simulink model "s0311_Bayesopt_SimulatorParameters"  (R2019b)
settings: Solver=FixedStepAuto  StartTime=0.0  StopTime=T_sim  FixedStep=dt  RelTol=1e-3
settings Model: Creator=paolo  LastModifiedBy=giaco
settings DebuggingCC: SFMachineParentedDataDiag=error

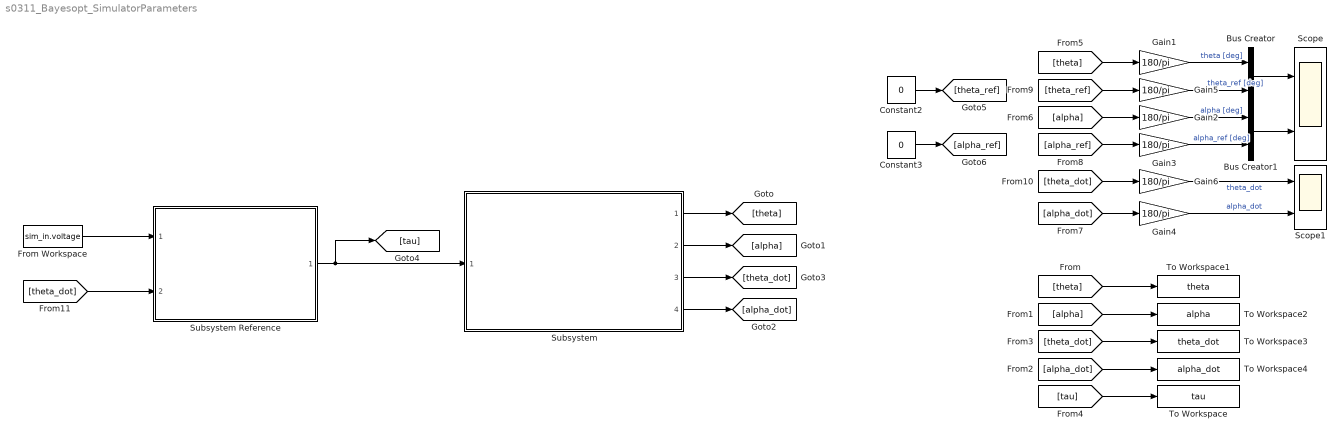
== system s0311_Bayesopt_SimulatorParameters ==
  Bus Creator : BusCreator  Inputs=2
  Bus Creator1 : BusCreator  Inputs=2
  Constant2 : Constant  Value=0
  Constant3 : Constant  Value=0
  From Workspace : FromWorkspace  VariableName=sim_in.voltage  SampleTime=0
  Gain{1..6} (6 alike) : Gain  Gain=180/pi
  Scope : Scope  NumInputPorts=2
  Scope1 : Scope  NumInputPorts=2
  Subsystem : Subsystem  ReferencedSubsystem=s0311_bayesopt_simulator  th_0=PARAMS.th_0  al_0=PARAMS.al_0  th_dot_0=PARAMS.th_dot_0  al_dot_0=PARAMS.al_dot_0
  Subsystem Reference : Subsystem  ReferencedSubsystem=s0303_motor_simulator  omega_0=PARAMS.th_dot_0  i_0=0
  To Workspace : ToWorkspace  VariableName=tau  SampleTime=-1
  To Workspace1 : ToWorkspace  VariableName=theta  SampleTime=-1
  To Workspace2 : ToWorkspace  VariableName=alpha  SampleTime=-1
  To Workspace3 : ToWorkspace  VariableName=theta_dot  SampleTime=-1
  To Workspace4 : ToWorkspace  VariableName=alpha_dot  SampleTime=-1
  wires:
  Subsystem/1 -> [theta]
  Subsystem/2 -> [alpha]
  Subsystem/4 -> [alpha_dot]
  Subsystem/3 -> [theta_dot]
  Subsystem Reference/1 -> Subsystem/1, [tau]
  From Workspace/1 -> Subsystem Reference/1
  [tau] -> To Workspace/1
  [theta] -> To Workspace1/1
  [alpha] -> To Workspace2/1
  [theta_dot] -> To Workspace3/1
  [alpha_dot] -> To Workspace4/1
  [theta] -> Gain1/1
  [alpha] -> Gain2/1
  [alpha_ref] -> Gain3/1
  [alpha_dot] -> Gain4/1
  Gain1/1 -> Bus Creator/1  "theta [deg]"
  [theta_ref] -> Gain5/1
  Gain5/1 -> Bus Creator/2  "theta_ref [deg]"
  Gain2/1 -> Bus Creator1/1  "alpha [deg]"
  Gain3/1 -> Bus Creator1/2  "alpha_ref [deg]"
  Constant2/1 -> [theta_ref]
  Constant3/1 -> [alpha_ref]
  [theta_dot] -> Gain6/1
  Bus Creator/1 -> Scope/1
  Bus Creator1/1 -> Scope/2
  [theta_dot] -> Subsystem Reference/2
  Gain4/1 -> Scope1/2  "alpha_dot"
  Gain6/1 -> Scope1/1  "theta_dot"
